simulink model "Battery_charge_discharge_FSBB_DCDC_constantCurrent_2020"  (R2020a)
settings: Solver=ode23tb  StartTime=0.0  StopTime=1.5  RelTol=1e-3  EnableMultiTasking=on
undefined symbols (not defined in the file or in its folder): Ion, Lithium
libraries: powerlib x21, powerlib_meascontrol x2, simulink x2, electricdrivelib x1
settings Model: Creator=Lei  LastModifiedBy=Loki
settings DataIOCC: LimitDataPoints=on  SaveFormat=Array  ReturnWorkspaceOutputs=off
settings OptimizationCC: LifeSpan=inf
settings DebuggingCC: SolverPrmCheckMsg=warning  SFUnexpectedBacktrackingDiag=warning  SFNoUnconditionalDefaultTransitionDiag=warning  SFExecutionAtInitializationDiag=none  ArithmeticOperatorsInVariantConditions=warning
settings HardwareCC: ProdBitPerPointer=32  ProdBitPerSizeT=32  ProdBitPerPtrDiffT=32  ProdLargestAtomicFloat=None  ProdIntDivRoundTo=Undefined  ProdEndianess=Unspecified  ProdWordSize=32  ProdHWDeviceType=32-bit Generic
settings ModelReferenceCC: PropagateSignalLabelsOutOfModel=off
settings SFSimCC: SimUseLocalCustomCode=off  CustomCodeUndefinedFunction=UseInterfaceOnly
settings RTWCC: RTWUseLocalCustomCode=off
settings CodeAppCC: StateflowObjectComments=on
settings GRTTargetCC: TargetLangStandard=C89/C90 (ANSI)
settings ConfigComp: CovMetricSettings=dw  CovSaveCumulativeToWorkspaceVar=on  CovSaveSingleToWorkspaceVar=on  CovExternalEMLEnable=off  CovSFcnEnable=off
settings SimscapeCC: SimscapeNormalizeSystem=off

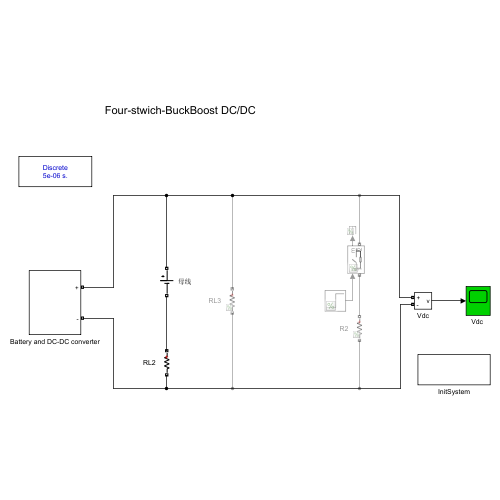
[thumbnail: Simulink's stored preview of the top-level diagram]
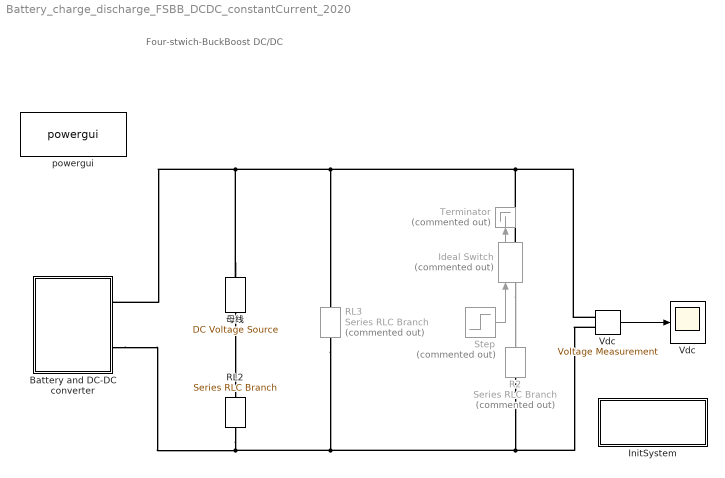
== system Battery_charge_discharge_FSBB_DCDC_constantCurrent_2020 ==
  note: Four-stwich-BuckBoost DC/DC
  Battery and DC-DC converter : Subsystem
  Ideal Switch : powerlib/Power Electronics/Ideal Switch  Commented=on  Ron=0.001  Lon=0  IC=0  Rs=1e5  Cs=inf  Measurements=on
  InitSystem : Subsystem
      settings: OpenFcn=Battery_charge_discharge_FSBB_param_init
  R2 : powerlib/Elements/Series RLC Branch  Commented=on  LConnTagsString=__new0  RConnTagsString=__new0  BranchType=R  Resistance=6  Inductance=1e-3  SetiL0=off  InitialCurrent=0  Capacitance=1e-6  Setx0=off  InitialVoltage=0  Measurements=None
  RL2 : powerlib/Elements/Series RLC Branch  LConnTagsString=__new0  RConnTagsString=__new0  BranchType=R  Resistance=0.315  Inductance=1e-3  SetiL0=off  InitialCurrent=0  Capacitance=1e-6  Setx0=off  InitialVoltage=0  Measurements=None
  RL3 : powerlib/Elements/Series RLC Branch  Commented=on  LConnTagsString=__new0  RConnTagsString=__new0  BranchType=R  Resistance=6  Inductance=1e-3  SetiL0=off  InitialCurrent=0  Capacitance=1e-6  Setx0=off  InitialVoltage=0  Measurements=None
  Step : Step  Commented=on  Time=0.3  After=3  SampleTime=0
  Terminator : Terminator  Commented=on
  Vdc : powerlib/Measurements/Voltage Measurement  PhasorSimulation=off  OutputType=Complex  PSBequivalent=0
  "Vdc " : Scope
  powergui : powerlib/powergui  Priority=1  SimulationMode=Discrete  SampleTime=5e-6  frequency=60  Iterations=50  frequencyindice=0  Pbase=100e6  ErrMax=1e-4  UnitsV=kV  UnitsW=MW  buscounter=0  FunctionMessages=off  echomessages=off  EnableUseOfTLC=off  CurrentSourceSwitches=off  DisableSnubberDevices=off  DisableRonSwitches=off  DisableVfSwitches=off  DisplayEquations=off  AutomaticDiscreteSolvers=off  SolverType=Tustin/Backward Euler (TBE)  Interpol=off  ExternalGateDelay=off  methode=off  Ts=100  x0status=blocks  SPID=off  SwTol=0  HookPort=off  NonlinearTolerance=1e-4  nMaxIteration=100  ContinueOnMaxIteration=off  RestoreLinks=warning  ResistiveCurrentMeasurement=off  Frange=[0:2:500]  Ylog=off  Xlog=on  ShowGrid=off  save=off  variable=ZData  structure=0  ZoomFFT=off  StartTime=0.0  cycles=1  DisplayStyle=1  fundamental=60  FreqAxis=off  MaxFrequency=1000  frequencyindicesteady=1  RmsSteady=1  display=off
  "母线  " : powerlib/Electrical Sources/DC Voltage Source  Amplitude=96  Measurements=None
  wires:
  Vdc/1 -> "Vdc "/1
  Step/1 -> Ideal Switch/1
  Ideal Switch/1 -> Terminator/1
  connections:
  Vdc/LConn1 -- Ideal Switch/RConn1 -- "母线  "/RConn1 -- Battery and DC-DC converter/RConn1 -- RL3/LConn1
  Vdc/LConn2 -- R2/RConn1 -- RL3/RConn1 -- RL2/RConn1 -- Battery and DC-DC converter/RConn2
  "母线  "/LConn1 -- RL2/LConn1
  Ideal Switch/LConn1 -- R2/LConn1

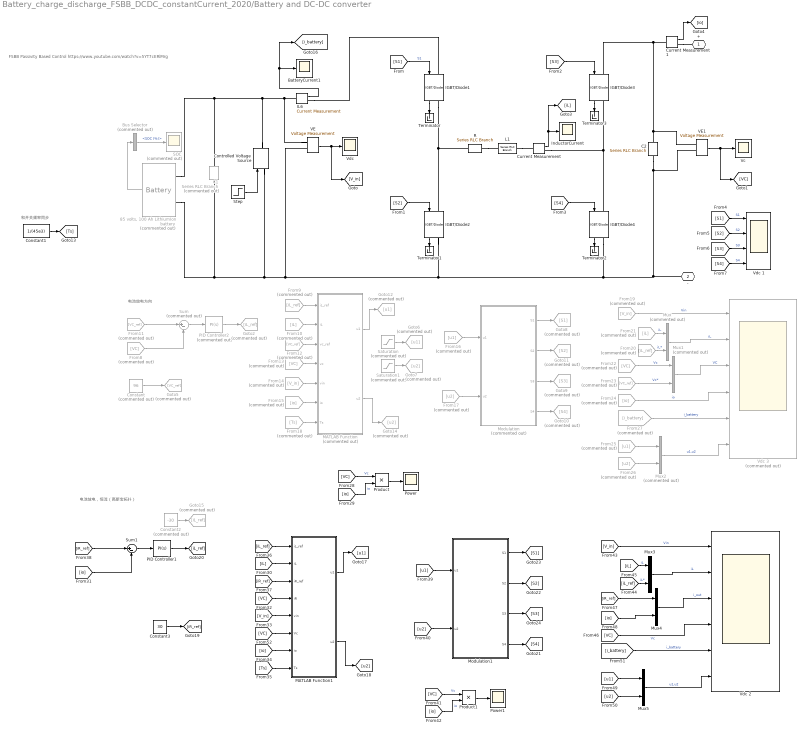
== system Battery_charge_discharge_FSBB_DCDC_constantCurrent_2020/Battery and DC-DC converter ==
  note: 电池放电，恒流（高斯宝拓扑）
  note: 电池放电方向
  note: 和开关频率同步
  note: FSBB Passivity Based Control
      | https://www.youtube.com/watch?v=5YT7cERlMrg
  "85 volts, 100 Ah LithiumIon battery " : electricdrivelib/Extra Sources/Battery  Commented=on  BatType=Lithium-Ion  ShowTempParam=off  ThermalPreset=no  ShowAgeParam=off  NomV=85  NomQ=100  SOC=80  Batt_Tr=30  PresetModel=off  MaxQ=107.6923  MinV=83.2  FullV=115.2  Dis_rate=20  R=0.0085  Normal_OP=96.1538  expZone="[92.2034           20]"  current=[6.5 13 32.5]  Units=Time  Tci=20  NomT=20  T2=-30  MaxQ2=4.8  FullV2=7.1  Normal_OP2=5.655  expZone2="[6.58           1]"  Rca=0.6  ti=2000  Dp=0  Neq0=0  Tsim=1e6  Ta1=25  Qeol=5.4*0.9  Reol=0.013333*1.2  Char_age=[2.3478, 3]  Dis_age=[2.3478, 10]  N1=1500  N2=10500  N3=1000  N4=1400  Ta2=45  N5=950
  BatteryCurrent1 : Scope
  Bus Selector : BusSelector  Commented=on  OutputSignals=SOC (%)
  C1 : powerlib/Elements/Series RLC Branch  Commented=on  LConnTagsString=__new0  RConnTagsString=__new0  BranchType=C  Resistance=5  Inductance=1e-3  SetiL0=off  InitialCurrent=0  Capacitance=1440e-6  Setx0=off  InitialVoltage=80  Measurements=None
  C2 : powerlib/Elements/Series RLC Branch  LConnTagsString=__new0  RConnTagsString=__new0  BranchType=C  Resistance=5  Inductance=1e-3  SetiL0=off  InitialCurrent=0  Capacitance=1440e-6  Setx0=off  InitialVoltage=80  Measurements=None
  Constant : Constant  Commented=on  Value=96
  Constant1 : Constant  Value=1/(45e3)
  Constant2 : Constant  Commented=on  Value=-30
  Constant3 : Constant  Value=30
  Controlled Voltage Source : powerlib/Electrical Sources/Controlled Voltage Source  Initialize=on  Source_Type=DC  Amplitude=98  Phase=0  Frequency=0  Measurements=None
  Current Measurement : powerlib/Measurements/Current Measurement  PhasorSimulation=off  OutputType=Complex  PSBequivalent=0
  Current Measurement1 : powerlib/Measurements/Current Measurement  PhasorSimulation=off  OutputType=Complex  PSBequivalent=0
  From10 : From  Commented=on  GotoTag=iL
  From11 : From  Commented=on  GotoTag=VC_ref
  From12 : From  Commented=on  GotoTag=VC_ref
  From13 : From  Commented=on  GotoTag=VC
  From14 : From  Commented=on  GotoTag=V_in
  From15 : From  Commented=on  GotoTag=io
  From16 : From  Commented=on  GotoTag=u1
  From17 : From  Commented=on  GotoTag=u2
  From18 : From  Commented=on  GotoTag=Ts
  From19 : From  Commented=on  GotoTag=V_in
  From20 : From  Commented=on  GotoTag=iL_ref
  From21 : From  Commented=on  GotoTag=iL
  From22 : From  Commented=on  GotoTag=VC
  From23 : From  Commented=on  GotoTag=VC_ref
  From24 : From  Commented=on  GotoTag=io
  From25 : From  Commented=on  GotoTag=u1
  From26 : From  Commented=on  GotoTag=u2
  From27 : From  Commented=on  GotoTag=i_battery
  From8 : From  Commented=on  GotoTag=VC
  From9 : From  Commented=on  GotoTag=iL_ref
  Goto10 : Goto  Commented=on  GotoTag=S4
  Goto11 : Goto  Commented=on  GotoTag=S2
  Goto12 : Goto  Commented=on  GotoTag=u1
  Goto14 : Goto  Commented=on  GotoTag=u2
  Goto15 : Goto  Commented=on  GotoTag=iL_ref
  Goto2 : Goto  Commented=on  GotoTag=iL_ref
  Goto5 : Goto  Commented=on  GotoTag=VC_ref
  Goto6 : Goto  Commented=on  GotoTag=u1
  Goto7 : Goto  Commented=on  GotoTag=u2
  Goto8 : Goto  Commented=on  GotoTag=S1
  Goto9 : Goto  Commented=on  GotoTag=S3
  IGBT/Diode{1..4} (4 alike) : powerlib/Power Electronics/IGBT//Diode  Ron=1e-3  Rs=1e5  Cs=inf  Measurements=on
  IL6 : powerlib/Measurements/Current Measurement  PhasorSimulation=off  OutputType=Complex  PSBequivalent=0
  InductorCurrent : Scope
  L1 : powerlib/Elements/Series RLC Branch  LConnTagsString=__new0  RConnTagsString=__new0  BranchType=L  Resistance=1.0  Inductance=20e-6  SetiL0=off  InitialCurrent=0  Capacitance=1.0  Setx0=off  InitialVoltage=0  Measurements=None
  MATLAB Function : MATLAB Function  Commented=on  TreatAsAtomicUnit=on
  MATLAB Function1 : MATLAB Function  TreatAsAtomicUnit=on
  Modulation : Subsystem  Commented=on
  Modulation1 : Subsystem
  Mux : Mux  Commented=on  Inputs=2
  Mux1 : Mux  Commented=on  Inputs=2
  Mux2 : Mux  Commented=on  Inputs=2
  Mux3 : Mux  Inputs=2
  Mux4 : Mux  Inputs=2
  Mux5 : Mux  Inputs=2
  PID Controller1 : simulink/Continuous/PID Controller  Controller=PI  Form=Parallel  TimeDomain=Continuous-time  UseExternalTs=off  SampleTime=-1  IntegratorMethod=Forward Euler  FilterMethod=Forward Euler  ControllerParametersSource=internal  P=15  I=1000  D=0  N=100  UseFilter=on  TunerSelectOption=Transfer Function Based (PID Tuner App)  InitialConditionSource=internal  InitialConditionForIntegrator=0  InitialConditionForFilter=0  DifferentiatorICPrevScaledInput=0  ExternalReset=none  TrackingMode=off  Kt=1  LimitOutput=on  UpperSaturationLimit=50  LowerSaturationLimit=-10  LinearizeAsGain=on  AntiWindupMode=none  Kb=1  POutMin=[]  POutMax=[]  IOutMin=[]  IOutMax=[]  DOutMin=[]  DOutMax=[]  NOutMin=[]  NOutMax=[]  SumOutMin=[]  SumOutMax=[]  SaturationOutMin=[]  SaturationOutMax=[]  PParamMin=[]  PParamMax=[]  IParamMin=[]  IParamMax=[]  DParamMin=[]  DParamMax=[]  NParamMin=[]  NParamMax=[]  KbParamMin=[]  KbParamMax=[]  KtParamMin=[]  KtParamMax=[]  KbOutMin=[]  KbOutMax=[]  KtOutMin=[]  KtOutMax=[]  IntegratorOutMin=[]  IntegratorOutMax=[]  FilterOutMin=[]  FilterOutMax=[]  SumI1OutMin=[]  SumI1OutMax=[]  SumI2OutMin=[]  SumI2OutMax=[]  SumI3OutMin=[]  SumI3OutMax=[]  SumI4OutMin=[]  SumI4OutMax=[]  SumDOutMin=[]  SumDOutMax=[]  DifferentiatorOutMin=[]  DifferentiatorOutMax=[]  FilterDiffOutCoefMin=[]  FilterDiffOutCoefMax=[]  ReciprocalOutMin=[]  ReciprocalOutMax=[]  SumDenOutMin=[]  SumDenOutMax=[]  SumNumOutMin=[]  SumNumOutMax=[]  DivideOutMin=[]  DivideOutMax=[]  UdiffTsProdOutMin=[]  UdiffTsProdOutMax=[]  NTsProdOutMin=[]  NTsProdOutMax=[]  UintegralTsProdOutMin=[]  UintegralTsProdOutMax=[]  UngainTsProdOutMin=[]  UngainTsProdOutMax=[]  IntegratorContinuousStateAttributes=''  IntegratorStateMustResolveToSignalObject=off  IntegratorRTWStateStorageClass=Auto  FilterContinuousStateAttributes=''  FilterStateMustResolveToSignalObject=off  FilterRTWStateStorageClass=Auto  ParallelPVariant=InternalParameters  IdealPVariant=Disabled  IVariant=InternalParameters  DVariant=Disabled  IntegratorVariant=Continuous  SatVariant=Enabled  AWVariant=Passthrough  PCopyVariant=Disabled  TRVariant=Disabled  FdbkBlocksVariant=Forward  IdealPFdbkVariant=Disabled  SatFdbkVariant=Disabled  DerivativeFilterVariant=Disabled  NVariant=Disabled  NCopyVariant=Disabled_SignalSpec  FilterICVariant=Disabled  IntegratorICVariant=InternalICs  ExternalResetVariant=Disabled  TRSumVariant=Passthrough  SumFdbkVariant=Disabled  SumVariant=Sum_PI  TsampFilterVariant=InternalTs  TsampNgainVariant=Passthrough  TsampIntegralVariant=Passthrough
  PID Controller2 : simulink/Continuous/PID Controller  Commented=on  Controller=PI  Form=Parallel  TimeDomain=Continuous-time  UseExternalTs=off  SampleTime=-1  IntegratorMethod=Forward Euler  FilterMethod=Forward Euler  ControllerParametersSource=internal  P=15  I=1000  D=0  N=100  UseFilter=on  TunerSelectOption=Transfer Function Based (PID Tuner App)  InitialConditionSource=internal  InitialConditionForIntegrator=0  InitialConditionForFilter=0  DifferentiatorICPrevScaledInput=0  ExternalReset=none  TrackingMode=off  Kt=1  LimitOutput=on  UpperSaturationLimit=50  LowerSaturationLimit=-10  LinearizeAsGain=on  AntiWindupMode=none  Kb=1  POutMin=[]  POutMax=[]  IOutMin=[]  IOutMax=[]  DOutMin=[]  DOutMax=[]  NOutMin=[]  NOutMax=[]  SumOutMin=[]  SumOutMax=[]  SaturationOutMin=[]  SaturationOutMax=[]  PParamMin=[]  PParamMax=[]  IParamMin=[]  IParamMax=[]  DParamMin=[]  DParamMax=[]  NParamMin=[]  NParamMax=[]  KbParamMin=[]  KbParamMax=[]  KtParamMin=[]  KtParamMax=[]  KbOutMin=[]  KbOutMax=[]  KtOutMin=[]  KtOutMax=[]  IntegratorOutMin=[]  IntegratorOutMax=[]  FilterOutMin=[]  FilterOutMax=[]  SumI1OutMin=[]  SumI1OutMax=[]  SumI2OutMin=[]  SumI2OutMax=[]  SumI3OutMin=[]  SumI3OutMax=[]  SumI4OutMin=[]  SumI4OutMax=[]  SumDOutMin=[]  SumDOutMax=[]  DifferentiatorOutMin=[]  DifferentiatorOutMax=[]  FilterDiffOutCoefMin=[]  FilterDiffOutCoefMax=[]  ReciprocalOutMin=[]  ReciprocalOutMax=[]  SumDenOutMin=[]  SumDenOutMax=[]  SumNumOutMin=[]  SumNumOutMax=[]  DivideOutMin=[]  DivideOutMax=[]  UdiffTsProdOutMin=[]  UdiffTsProdOutMax=[]  NTsProdOutMin=[]  NTsProdOutMax=[]  UintegralTsProdOutMin=[]  UintegralTsProdOutMax=[]  UngainTsProdOutMin=[]  UngainTsProdOutMax=[]  IntegratorContinuousStateAttributes=''  IntegratorStateMustResolveToSignalObject=off  IntegratorRTWStateStorageClass=Auto  FilterContinuousStateAttributes=''  FilterStateMustResolveToSignalObject=off  FilterRTWStateStorageClass=Auto  ParallelPVariant=InternalParameters  IdealPVariant=Disabled  IVariant=InternalParameters  DVariant=Disabled  IntegratorVariant=Continuous  SatVariant=Enabled  AWVariant=Passthrough  PCopyVariant=Disabled  TRVariant=Disabled  FdbkBlocksVariant=Forward  IdealPFdbkVariant=Disabled  SatFdbkVariant=Disabled  DerivativeFilterVariant=Disabled  NVariant=Disabled  NCopyVariant=Disabled_SignalSpec  FilterICVariant=Disabled  IntegratorICVariant=InternalICs  ExternalResetVariant=Disabled  TRSumVariant=Passthrough  SumFdbkVariant=Disabled  SumVariant=Sum_PI  TsampFilterVariant=InternalTs  TsampNgainVariant=Passthrough  TsampIntegralVariant=Passthrough
  Power : Scope
  Power1 : Scope
  Product : Product
  Product1 : Product
  R : powerlib/Elements/Series RLC Branch  LConnTagsString=__new0  RConnTagsString=__new0  BranchType=R  Resistance=0.004  Inductance=1e-3  SetiL0=off  InitialCurrent=0  Capacitance=1e-3  Setx0=off  InitialVoltage=80  Measurements=None
  SOC : Scope  Commented=on
  Saturation : Saturate  Commented=on  UpperLimit=1  LowerLimit=-1  LinearizeAsGain=off
  Saturation1 : Saturate  Commented=on  UpperLimit=1  LowerLimit=-1  LinearizeAsGain=off
  Step : Step  Time=0.7  Before=102.5  After=93  SampleTime=0
  Sum : Sum  Commented=on  Inputs=|+-
  Sum1 : Sum  Inputs=|+-
  Terminator{,1..3} (4 alike) : Terminator
  VE : powerlib/Measurements/Voltage Measurement  PhasorSimulation=off  OutputType=Complex  PSBequivalent=0
  VE1 : powerlib/Measurements/Voltage Measurement  PhasorSimulation=off  OutputType=Complex  PSBequivalent=0
  Vc : Scope
  "Vdc " : Scope
  Vdc 1 : Scope  NumInputPorts=4
  Vdc 2 : Scope  NumInputPorts=6
  Vdc 3 : Scope  Commented=on  NumInputPorts=6
  + : PMIOPort  Tag=PMCPort  Side=Right
  - : PMIOPort  Tag=PMCPort  Port=2  Side=Right
  wires:
  VE/1 -> [V_in], "Vdc "/1
  IL6/1 -> BatteryCurrent1/1, [i_battery]
  Bus Selector/1 -> SOC/1  "<SOC (%)>"
  "85 volts, 100 Ah LithiumIon battery "/1 -> Bus Selector/1
  [S2] -> IGBT/Diode2/1
  [S1] -> IGBT/Diode1/1  "S1"
  [S1] -> Vdc 1/1  "S1"
  [S2] -> Vdc 1/2  "S2"
  [S3] -> Vdc 1/3  "S3"
  [S4] -> Vdc 1/4  "S4"
  Current Measurement/1 -> [iL], InductorCurrent/1
  [S3] -> IGBT/Diode3/1
  [S4] -> IGBT/Diode4/1
  Sum/1 -> PID Controller2/1
  PID Controller2/1 -> Goto2/1
  Current Measurement1/1 -> [io]
  From9/1 -> MATLAB Function/1(iL_ref)
  From10/1 -> MATLAB Function/2(iL)
  From12/1 -> MATLAB Function/3(vc_ref)
  From13/1 -> MATLAB Function/4(vc)
  From14/1 -> MATLAB Function/5(vin)
  From18/1 -> MATLAB Function/7(Ts)
  From15/1 -> MATLAB Function/6(io)
  Saturation/1 -> Goto6/1
  Saturation1/1 -> Goto7/1
  From16/1 -> Modulation/1(u1)
  From17/1 -> Modulation/2(u2)
  Modulation/1(S1) -> Goto8/1
  Modulation/3(S3) -> Goto9/1
  Modulation/4(S4) -> Goto10/1
  Modulation/2(S2) -> Goto11/1
  Constant1/1 -> [Ts]
  From19/1 -> Vdc 3/1  "Vin"
  Mux/1 -> Vdc 3/2  "iL"
  From20/1 -> Mux/2  "iL*"
  From21/1 -> Mux/1  "iL"
  From22/1 -> Mux1/1  "Vc"
  From23/1 -> Mux1/2  "Vc*"
  Mux1/1 -> Vdc 3/3  "VC"
  Mux2/1 -> Vdc 3/6  "u1,u2"
  From25/1 -> Mux2/1
  From26/1 -> Mux2/2
  IGBT/Diode1/1 -> Terminator/1
  IGBT/Diode2/1 -> Terminator1/1
  IGBT/Diode4/1 -> Terminator2/1
  IGBT/Diode3/1 -> Terminator3/1
  VE1/1 -> [VC], Vc/1
  Step/1 -> Controlled Voltage Source/1
  MATLAB Function/2(u2) -> Goto14/1
  MATLAB Function/1(u1) -> Goto12/1
  Constant2/1 -> Goto15/1
  From24/1 -> Vdc 3/4  "io"
  From27/1 -> Vdc 3/5  "i_battery"
  From11/1 -> Sum/1
  [VC] -> Product/1  "Vc"
  [io] -> Product/2  "io"
  Product/1 -> Power/1
  Constant/1 -> Goto5/1
  From8/1 -> Sum/2
  [io] -> MATLAB Function1/7(io)
  [iL] -> MATLAB Function1/2(iL)
  [VC] -> MATLAB Function1/4(iR)
  [iL_ref] -> MATLAB Function1/1(iL_ref)
  [iR_ref] -> MATLAB Function1/3(iR_ref)
  [V_in] -> MATLAB Function1/5(vin)
  MATLAB Function1/1(u1) -> [u1]
  [Ts] -> MATLAB Function1/8(Ts)
  MATLAB Function1/2(u2) -> [u2]
  Constant3/1 -> [iR_ref]
  [iR_ref] -> Sum1/1
  Sum1/1 -> PID Controller1/1
  [io] -> Sum1/2
  PID Controller1/1 -> [iL_ref]
  [VC] -> Product1/1  "Vc"
  Modulation1/4(S4) -> [S4]
  Modulation1/1(S1) -> [S1]
  [u2] -> Modulation1/2(u2)
  Modulation1/2(S2) -> [S2]
  Modulation1/3(S3) -> [S3]
  [io] -> Product1/2  "io"
  [u1] -> Modulation1/1(u1)
  Product1/1 -> Power1/1
  [iL_ref] -> Mux3/2  "iL*"
  [u1] -> Mux5/1
  Mux5/1 -> Vdc 2/6  "u1,u2"
  [V_in] -> Vdc 2/1  "Vin"
  [i_battery] -> Vdc 2/5  "i_battery"
  Mux4/1 -> Vdc 2/3  "i_out"
  Mux3/1 -> Vdc 2/2  "iL"
  [iL] -> Mux3/1  "iL"
  [u2] -> Mux5/2
  [VC] -> Vdc 2/4  "Vc"
  [iR_ref] -> Mux4/1
  [io] -> Mux4/2
  [VC] -> MATLAB Function1/6(Vc)
  connections:
  VE1/LConn2 -- C2/RConn1 -- -/RConn1 -- IGBT/Diode4/RConn1 -- VE/LConn2 -- C1/RConn1 -- "85 volts, 100 Ah LithiumIon battery "/LConn2 -- Controlled Voltage Source/LConn1 -- IGBT/Diode2/RConn1
  C2/LConn1 -- IGBT/Diode3/LConn1 -- Current Measurement1/LConn1 -- VE1/LConn1
  VE/LConn1 -- "85 volts, 100 Ah LithiumIon battery "/LConn1 -- C1/LConn1 -- Controlled Voltage Source/RConn1 -- IL6/LConn1
  IL6/RConn1 -- IGBT/Diode1/LConn1
  IGBT/Diode1/RConn1 -- R/RConn1 -- IGBT/Diode2/LConn1
  Current Measurement/RConn1 -- IGBT/Diode4/LConn1 -- IGBT/Diode3/RConn1
  L1/RConn1 -- Current Measurement/LConn1
  R/LConn1 -- L1/LConn1
  Current Measurement1/RConn1 -- +/RConn1

== system Battery_charge_discharge_FSBB_DCDC_constantCurrent_2020/InitSystem ==

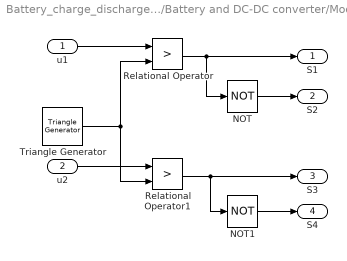
== system Battery_charge_discharge_FSBB_DCDC_constantCurrent_2020/Battery and DC-DC converter/Modulation ==
  u1 : Inport
  u2 : Inport  Port=2
  NOT : Logic  Operator=NOT  AllPortsSameDT=off  OutDataTypeStr=boolean
  NOT1 : Logic  Operator=NOT  AllPortsSameDT=off  OutDataTypeStr=boolean
  Relational Operator : RelationalOperator  Operator=>  OutDataTypeStr=boolean  RndMeth=Simplest
  Relational Operator1 : RelationalOperator  Operator=>  OutDataTypeStr=boolean  RndMeth=Simplest
  Triangle Generator : powerlib_meascontrol/Pulse & Signal Generators/Triangle Generator  Freq=45e3  Phase=0  Ts=0
  S1 : Outport
  S2 : Outport  Port=2
  S3 : Outport  Port=3
  S4 : Outport  Port=4
  wires:
  u1/1 -> Relational Operator/1
  Triangle Generator/1 -> Relational Operator1/2, Relational Operator/2
  u2/1 -> Relational Operator1/1
  Relational Operator/1 -> NOT/1, S1/1
  NOT/1 -> S2/1
  Relational Operator1/1 -> NOT1/1, S3/1
  NOT1/1 -> S4/1

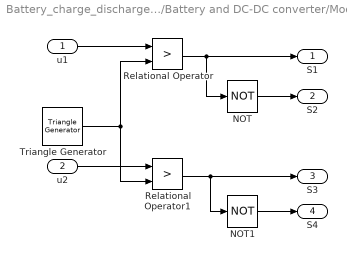
== system Battery_charge_discharge_FSBB_DCDC_constantCurrent_2020/Battery and DC-DC converter/Modulation1 ==
  u1 : Inport
  u2 : Inport  Port=2
  NOT : Logic  Operator=NOT  AllPortsSameDT=off  OutDataTypeStr=boolean
  NOT1 : Logic  Operator=NOT  AllPortsSameDT=off  OutDataTypeStr=boolean
  Relational Operator : RelationalOperator  Operator=>  OutDataTypeStr=boolean  RndMeth=Simplest
  Relational Operator1 : RelationalOperator  Operator=>  OutDataTypeStr=boolean  RndMeth=Simplest
  Triangle Generator : powerlib_meascontrol/Pulse & Signal Generators/Triangle Generator  Freq=45e3  Phase=0  Ts=0
  S1 : Outport
  S2 : Outport  Port=2
  S3 : Outport  Port=3
  S4 : Outport  Port=4
  wires:
  u1/1 -> Relational Operator/1
  Triangle Generator/1 -> Relational Operator1/2, Relational Operator/2
  u2/1 -> Relational Operator1/1
  Relational Operator/1 -> NOT/1, S1/1
  NOT/1 -> S2/1
  Relational Operator1/1 -> NOT1/1, S3/1
  NOT1/1 -> S4/1

== matlab function Battery_charge_discharge_FSBB_DCDC_constantCurrent_2020/Battery and DC-DC converter/MATLAB Function1 ==
  settings: updateMethod=DISCRETE
  data: iL_ref input; u1 output; iL input; iR_ref input; iR input; vin input; Vc input; io input; Ts input; u2 output
function [u1, u2] = Passivity_BC(iL_ref, iL,iR_ref, iR, vin, Vc,io, Ts)
%% system parameters
L = 20e-6;  % Inductance 电感 20uH
RL = 0.004;
Co = 1440e-6;  % 电容大小
R = Vc/io;  % 负载等效电阻

zeta1 = 6;  % dumping gains
zeta2 = 0.08; 

% error functions: state variable
x1 = iL - iL_ref;
x2 = iR - iR_ref;
persistent iL_ref_old iR_ref_old;
if isempty(iL_ref_old)
    iL_ref_old = 0;
    iR_ref_old = 0;
end

diL_ref = (iL_ref - iL_ref_old) / Ts;
diR_ref = (iR_ref - iR_ref_old) / Ts;
%% calculate switching signal: u1,u2
u2 = 1 / iL_ref * (iL_ref - diR_ref * Co * R - iR_ref + x2*zeta2);
u1 = 1 / vin * (L*diL_ref + RL*iL_ref + iR_ref * R * (1-u2) - x1*zeta1);

iL_ref_old = iL_ref;
iR_ref_old = iR_ref;

== matlab function Battery_charge_discharge_FSBB_DCDC_constantCurrent_2020/Battery and DC-DC converter/MATLAB Function ==
  settings: updateMethod=DISCRETE
  data: iL_ref input; u1 output; iL input; vc_ref input; vc input; vin input; io input; Ts input; u2 output
function [u1, u2] = Passivity_BC(iL_ref, iL, vc_ref, vc, vin, io, Ts)
%% system parameters
L = 20e-6;  % Inductance 电感 20uH
RL = 0.004;
Co = 1440e-6;  % 电容大小
R = vc_ref/io;  % 负载等效电阻

zeta1 = 6;  % dumping gains
zeta2 = 0.08; 

% error functions: state variable
x1 = iL - iL_ref;
x2 = vc - vc_ref;
persistent iL_ref_old vc_ref_old;
if isempty(iL_ref_old)
    iL_ref_old = 0;
    vc_ref_old = 0;
end

diL_ref = (iL_ref - iL_ref_old) / Ts;
dvc_ref = (vc_ref - vc_ref_old) / Ts;
%% calculate switching signal: u1,u2
u2 = 1 / iL_ref * (iL_ref - dvc_ref * Co - vc_ref/R + x2*zeta2);
u1 = 1 / vin * (L*diL_ref + RL*iL_ref + vc_ref*(1-u2) - x1*zeta1);
iL_ref_old = iL_ref;
vc_ref_old = vc_ref;
